simulink model "RC_Triggering"  (R2024a)
settings: Solver=VariableStepAuto  StartTime=0.0  StopTime=0.08  RelTol=1e-3
libraries: spsVoltageMeasurementLib x5, spsSeriesRLCBranchLib x3, spsDiodeLib x2, spsACVoltageSourceLib x1, spsThyristorLib x1, sps_lib x1
settings Model: Creator=bhavi  LastModifiedBy=bhavi

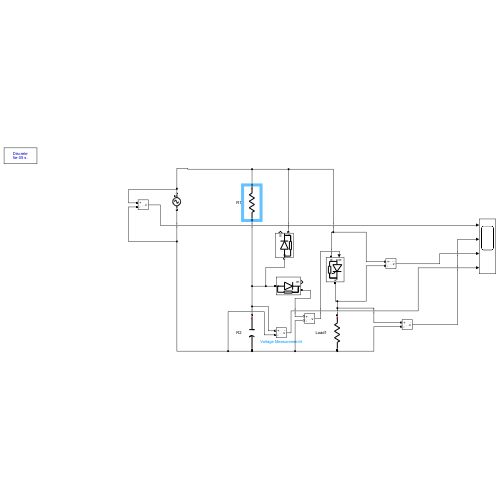
[thumbnail: Simulink's stored preview of the top-level diagram]
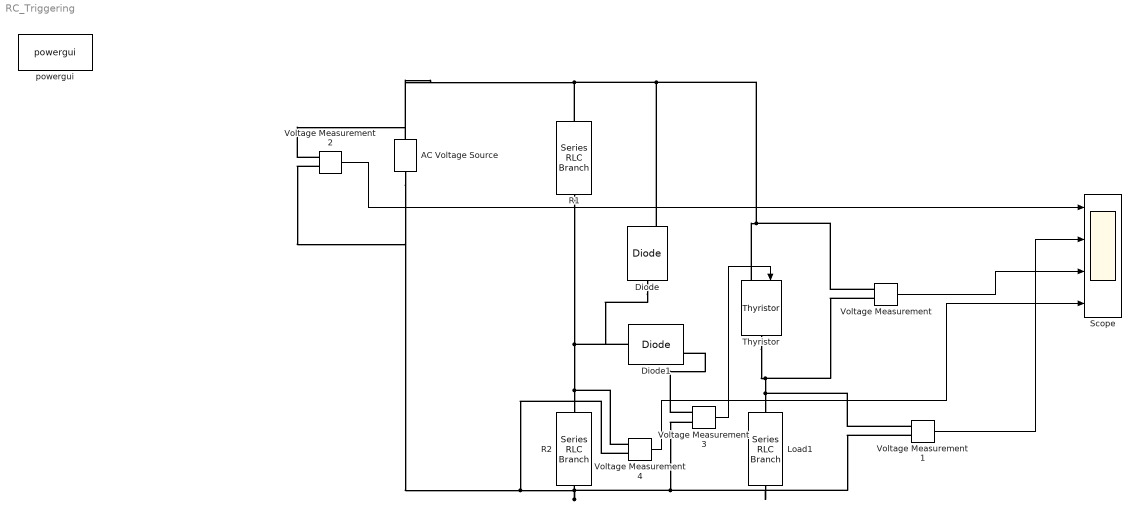
== system RC_Triggering ==
  AC Voltage Source : spsACVoltageSourceLib/AC Voltage Source  Amplitude=100  Phase=0  Frequency=50  SampleTime=0  Measurements=None  BusType=swing  Pref=10e3  Qref=0  Qmin=-inf  Qmax=+inf
  Diode : spsDiodeLib/Diode  Ron=0.001  Lon=0  Vf=0.8  IC=0  UseSnubber=0  Rs=500  Cs=0.1e-9  Measurements=on
  Diode1 : spsDiodeLib/Diode  Ron=0.001  Lon=0  Vf=0.8  IC=0  UseSnubber=0  Rs=500  Cs=0.1e-9  Measurements=on
  Load1 : spsSeriesRLCBranchLib/Series RLC Branch  LConnTagsString=__new0  RConnTagsString=__new0  BranchType=R  Resistance=100  Inductance=0  SetiL0=off  InitialCurrent=0  Capacitance=0  Setx0=off  InitialVoltage=0  Measurements=None
  R1 : spsSeriesRLCBranchLib/Series RLC Branch  LConnTagsString=__new0  RConnTagsString=__new0  BranchType=R  Resistance=30000  Inductance=0  SetiL0=off  InitialCurrent=0  Capacitance=0  Setx0=off  InitialVoltage=0  Measurements=None
  R2 : spsSeriesRLCBranchLib/Series RLC Branch  LConnTagsString=__new0  RConnTagsString=__new0  BranchType=C  Resistance=500  Inductance=0  SetiL0=off  InitialCurrent=0  Capacitance=0.1e-6  Setx0=off  InitialVoltage=0  Measurements=None
  Scope : Scope  NumInputPorts=4
  Thyristor : spsThyristorLib/Thyristor  Ron=0.001  Lon=0  Vf=0.6  IC=0  Rs=0  Cs=250e-9  Measurements=off
  Voltage Measurement{,1..4} (5 alike) : spsVoltageMeasurementLib/Voltage Measurement  PhasorSimulation=off  OutputType=Complex  PSBequivalent=0
  powergui : sps_lib/powergui  Priority=1  SimulationMode=Discrete  SampleTime=50e-6  frequency=60  Iterations=50  frequencyindice=50  Pbase=100e6  ErrMax=1e-4  UnitsV=kV  UnitsW=MW  buscounter=0  FunctionMessages=off  echomessages=off  EnableUseOfTLC=off  CurrentSourceSwitches=off  DisableSnubberDevices=off  DisableRonSwitches=off  DisableVfSwitches=off  DisplayEquations=off  AutomaticDiscreteSolvers=off  SolverType=Tustin/Backward Euler (TBE)  Interpol=off  ExternalGateDelay=off  methode=off  Ts=100  x0status=blocks  SPID=on  SwTol=0  HookPort=off  NonlinearTolerance=1e-4  nMaxIteration=100  ContinueOnMaxIteration=off  RestoreLinks=warning  ResistiveCurrentMeasurement=off  Frange=[0:2:500]  Ylog=off  Xlog=on  ShowGrid=off  save=off  variable=ZData  structure=0  ZoomFFT=off  StartTime=0.0  cycles=1  DisplayStyle=1  fundamental=60  FreqAxis=off  MaxFrequency=1000  frequencyindicesteady=1  RmsSteady=1  display=off
  wires:
  Voltage Measurement1/1 -> Scope/2
  Voltage Measurement/1 -> Scope/3
  Voltage Measurement2/1 -> Scope/1
  Voltage Measurement3/1 -> Thyristor/1
  Voltage Measurement4/1 -> Scope/4
  connections:
  R2/RConn1 -- Voltage Measurement3/LConn2 -- Voltage Measurement1/LConn2 -- Load1/RConn1 -- Voltage Measurement4/LConn2 -- Voltage Measurement2/LConn2 -- AC Voltage Source/LConn1
  Thyristor/LConn1 -- Voltage Measurement/LConn1 -- Diode/RConn1 -- AC Voltage Source/RConn1 -- Voltage Measurement2/LConn1 -- R1/LConn1
  Voltage Measurement/LConn2 -- Thyristor/RConn1 -- Voltage Measurement1/LConn1 -- Load1/LConn1
  R1/RConn1 -- Diode/LConn1 -- Diode1/LConn1 -- Voltage Measurement4/LConn1 -- R2/LConn1
  Voltage Measurement3/LConn1 -- Diode1/RConn1
